simulink model "pressure"  (R2020b)
settings: Solver=VariableStepAuto  StartTime=0.0  StopTime=10.0  RelTol=1e-3
model mask{scale=1, bias=0, noise=0, p_sath=inf, p_satl=-inf, sample_rate=2000}
  mask prompts: scale "Scale Factor:"; bias "Bias [Pa]:"; noise "Noise [Pa]:"; p_sath "Upper limit [Pa]:"; p_satl "Lower limit [Pa]:"; sample_rate "Sample Rate [Hz]:"
model workspace (MAT data in the model file):
  bias = Simulink.Parameter
  bias.Value = 0
  bias.DataType = 'auto'
  bias.Dimensions = [1 1]
  noise = Simulink.Parameter
  noise.Value = 0
  noise.DataType = 'auto'
  noise.Dimensions = [1 1]
  p_sath = Simulink.Parameter
  p_sath.Value = Inf
  p_sath.DataType = 'auto'
  p_sath.Dimensions = [1 1]
  p_satl = Simulink.Parameter
  p_satl.Value = -Inf
  p_satl.DataType = 'auto'
  p_satl.Dimensions = [1 1]
  sample_rate = Simulink.Parameter
  sample_rate.Value = 2000
  sample_rate.DataType = 'auto'
  sample_rate.Dimensions = [1 1]
  scale = Simulink.Parameter
  scale.Value = 1
  scale.DataType = 'auto'
  scale.Dimensions = [1 1]
undefined symbols (not defined in the file): psat_l
libraries: simulink x1
settings Model: ParameterArgumentNames=bias,noise,p_sath,p_satl,sample_rate,scale  OrderedModelArguments=off  Creator=brian  LastModifiedBy=brian

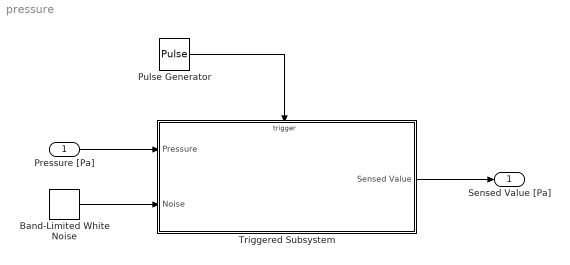
== system pressure ==
  Pressure [Pa] : Inport
  Band-Limited White Noise : simulink/Sources/Band-Limited White Noise  Cov=noise  Ts=0.1  seed=[23341]
  Pulse Generator : DiscretePulseGenerator  PulseType=Time based  Period=1/sample_rate  PulseWidth=5
  Triggered Subsystem : Subsystem  TreatAsAtomicUnit=on
  Sensed Value [Pa] : Outport
  wires:
  Pulse Generator/1 -> Triggered Subsystem/Trigger
  Pressure [Pa]/1 -> Triggered Subsystem/1(Pressure)
  Band-Limited White Noise/1 -> Triggered Subsystem/2(Noise)
  Triggered Subsystem/1(Sensed Value) -> Sensed Value [Pa]/1

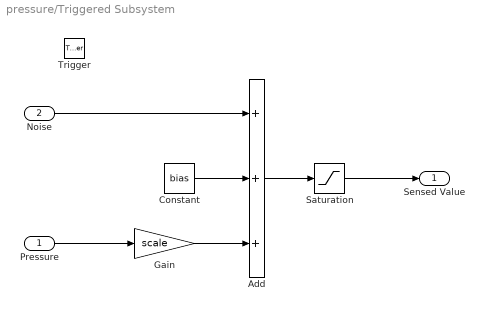
== system pressure/Triggered Subsystem ==
  Pressure : Inport
  Noise : Inport  Port=2
  Trigger : TriggerPort  VariantControl=Variant
  Add : Sum  Inputs=+++
  Constant : Constant  Value=bias
  Gain : Gain  Gain=scale
  Saturation : Saturate  UpperLimit=p_sath  LowerLimit=psat_l
  Sensed Value : Outport
  wires:
  Pressure/1 -> Gain/1
  Constant/1 -> Add/2
  Noise/1 -> Add/1
  Gain/1 -> Add/3
  Add/1 -> Saturation/1
  Saturation/1 -> Sensed Value/1
